simulink model "rst_auto_reg_test"  (R2019a)
settings: Solver=VariableStepAuto  StartTime=0.0  StopTime=150  RelTol=1e-3
values from neighbouring files (symbols this model uses):
  A = den    [cod_teste_RST_2.m]
  B = num    (= 1)    [cod_teste_RST_2.m]
  den = [10 1]    [cod_teste_RST_1.m]    (also in cod_teste_RST_2.m = [0.1 1.1 1])
  ep = 0.6    [cod_teste_RST_2.m]
  num = 1    [cod_teste_RST_1.m]    (also in cod_teste_RST_2.m)
  R = X(1)    [cod_teste_RST_1.m]    (also in cod_teste_RST_2.m = [X(1) X(2)])
  S = X(2:end)    [cod_teste_RST_1.m]    (also in cod_teste_RST_2.m = [X(3) X(4)])
  T = sum(PMF)/sum(B)    [cod_teste_RST_1.m]    (also in cod_teste_RST_2.m = sum(Am)/sum(B))
  Ta = 1    [cod_teste_RST_1.m]    (also in cod_teste_RST_2.m = 0.1)
  Ts = 1    [cod_teste_RST_2.m]
libraries: dspinverses x2
settings Model: Creator=Carlos Henrique  LastModifiedBy=PICHAU
settings DataIOCC: SaveOutput=off  SaveState=on  SignalLogging=off  DSMLogging=off  ReturnWorkspaceOutputs=off
settings DebuggingCC: ArithmeticOperatorsInVariantConditions=warning

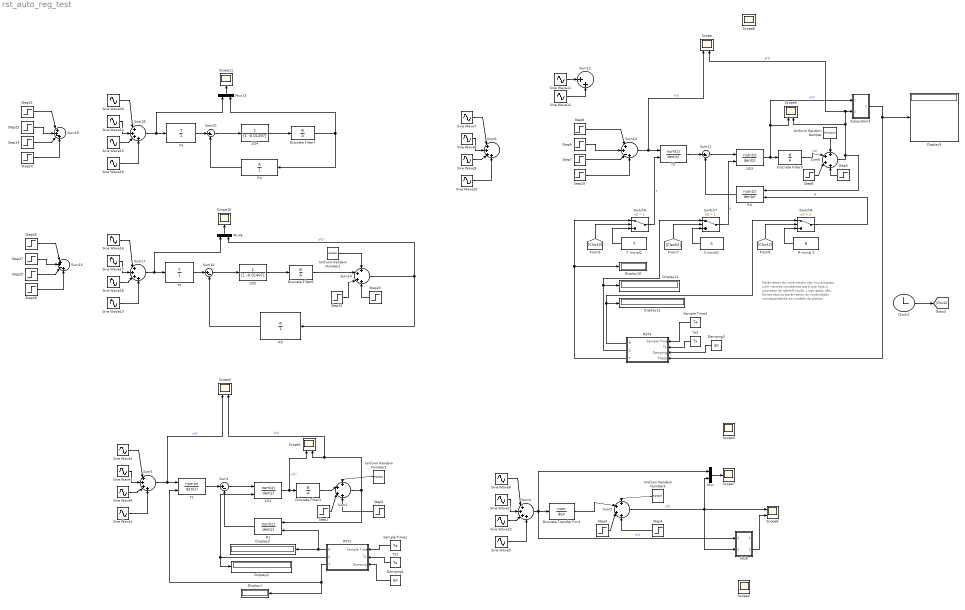
== system rst_auto_reg_test ==
  note: Parâmetros do controlador são inicializados
      | com valores constantes para que haja o
      | processo de identificação. Logo após, são
      | fornecidos os parâmetros do controlador
      | correspondente ao modelo da planta.
  1/S1 : DiscreteFilter  Numerator=1  DenominatorSource=Input port  Denominator=1  a0EqualsOne=on
      settings: InputPortMap=u0,p3
  1/S3 : DiscreteFilter  Numerator=1  DenominatorSource=Input port  Denominator=1  a0EqualsOne=on
      settings: InputPortMap=u0,p3
  1/S4 : DiscreteFilter  Numerator=1  Denominator=[1 -0.01497]  a0EqualsOne=on
  1/S5 : DiscreteFilter  Numerator=1  Denominator=[1 -0.01497]  a0EqualsOne=on
  Clock2 : Clock
  Damping1 : Constant  Value=ep
  Damping3 : Constant  Value=ep
  Discrete Transfer Fcn2 : DiscreteTransferFcn  Numerator=num  Denominator=den  SampleTime=Ta
  Discrete Filter{1,3,6..7} (4 alike) : DiscreteFilter  Numerator=B  Denominator=A  SampleTime=0.1  a0EqualsOne=on
  Display{1..3,9..12} (7 alike) : Display
  MQR : Subsystem
  Mux : Mux  Inputs=2
  Mux13 : Mux  Inputs=2
  Mux8 : Mux  Inputs=2
  R inicial 2 : Constant  Value=R
  R1 : DiscreteFilter  NumeratorSource=Input port  Numerator=[-620.2 131.3]  Denominator=1
      settings: InputPortMap=u0,p1
  R3 : DiscreteFilter  NumeratorSource=Input port  Numerator=[-620.2 131.3]  Denominator=1
      settings: InputPortMap=u0,p1
  R4 : DiscreteFilter  Numerator=R  Denominator=1
  R5 : DiscreteFilter  Numerator=R  Denominator=1
  RST1 : Subsystem
  RST3 : Subsystem
  S inicial2 : Constant  Value=S
  Sample Time1 : Constant  Value=Ta
  Sample Time3 : Constant  Value=Ta
  Scope{,1..2,4,6,8..9} (7 alike) : Scope  NumInputPorts=2
  Scope{3,7,10..11} (4 alike) : Scope
  Sine Wave{1,5,10,13,19} (5 alike) : Sin  Frequency=8  SampleTime=0
  Sine Wave{2,6..7,11,16,20} (6 alike) : Sin  SampleTime=0
  Sine Wave{3,8,12,14,17,21} (6 alike) : Sin  Frequency=2  SampleTime=0
  Sine Wave{4,9,15,18,22} (5 alike) : Sin  Frequency=4  SampleTime=0
  Step1 : Step  Time=50  SampleTime=0
  Step10 : Step  Time=30  SampleTime=0
  Step13 : Step  Time=50  SampleTime=0
  Step14 : Step  Time=20  After=2  SampleTime=0
  Step2 : Step  Time=51  After=-1  SampleTime=0
  Step21 : Step  Time=0  SampleTime=0
  Step22 : Step  Time=10  After=3  SampleTime=0
  Step23 : Step  Time=51  After=-1  SampleTime=0
  Step24 : Step  Time=30  SampleTime=0
  Step25 : Step  Time=20  After=2  SampleTime=0
  Step26 : Step  Time=0  SampleTime=0
  Step27 : Step  Time=10  After=3  SampleTime=0
  Step28 : Step  Time=30  SampleTime=0
  Step3 : Step  Time=50  SampleTime=0
  Step4 : Step  Time=51  After=-1  SampleTime=0
  Step5 : Step  Time=51  After=-0.2  SampleTime=0
  Step6 : Step  Time=50  After=0.2  SampleTime=0
  Step7 : Step  Time=20  After=2  SampleTime=0
  Step8 : Step  Time=0  SampleTime=0
  Step9 : Step  Time=10  After=3  SampleTime=0
  Subsystem3 : Subsystem
  Sum{1,11,16,20} (4 alike) : Sum  Inputs=|+-
  Sum10 : Sum  Inputs=|++-+
  Sum12 : Sum  Inputs=|++
  Sum{2,5..6,14} (4 alike) : Sum  Inputs=++++
  Sum15 : Sum  Inputs=|++-+
  Sum{3..4,9,17..18} (5 alike) : Sum  Inputs=|++++
  Sum19 : Sum  Inputs=|++-+
  Switch6 : Switch  Criteria=u2 > Threshold  Threshold=1
  Switch7 : Switch  Criteria=u2 > Threshold  Threshold=1
  Switch8 : Switch  Criteria=u2 > Threshold  Threshold=1
  T inicial2 : Constant  Value=T
  T1 : DiscreteFilter  NumeratorSource=Input port  Numerator=13.39  Denominator=1
      settings: InputPortMap=u0,p1
  T3 : DiscreteFilter  NumeratorSource=Input port  Numerator=13.39  Denominator=1
      settings: InputPortMap=u0,p1
  T4 : DiscreteFilter  Numerator=T  Denominator=1  a0EqualsOne=on
  T5 : DiscreteFilter  Numerator=T  Denominator=1  a0EqualsOne=on
  Ts1 : Constant  Value=Ts
  Ts3 : Constant  Value=Ts
  Uniform Random Number : UniformRandomNumber  Minimum=-0.01  Maximum=0.01  SampleTime=0
  Uniform Random Number1 : UniformRandomNumber  Minimum=-0.1  Maximum=0.1  SampleTime=0
  Uniform Random Number2 : UniformRandomNumber  Minimum=-0.1  Maximum=0.1  SampleTime=0
  Uniform Random Number3 : UniformRandomNumber  Minimum=-0.01  Maximum=0.01  SampleTime=0
  wires:
  Sine Wave10/1 -> Sum9/4
  Ts3/1 -> RST3/2(Ts)
  T3/1 -> Sum11/1
  R3/1 -> Sum11/2
  RST3/1(R) -> Switch8/1, Display12/1
  Switch8/1 -> R3/2  "R"
  Step7/1 -> Sum10/3
  RST3/2(S) -> Switch7/1, Display11/1
  [Clock2] -> Switch7/2
  Subsystem3/1(Out1) -> RST3/4(Theta), Display9/1
  T inicial2/1 -> Switch6/3
  Sine Wave7/1 -> Sum9/1
  Clock2/1 -> [Clock2]
  S inicial2/1 -> Switch7/3
  Sum11/1 -> 1/S3/1
  Switch6/1 -> T3/2  "T"
  [Clock2] -> Switch6/2
  Switch7/1 -> 1/S3/2  "S"
  Sample Time3/1 -> RST3/1(Sample Time)
  Sine Wave8/1 -> Sum9/2
  Damping3/1 -> RST3/3(Damping)
  RST3/3(T) -> Switch6/1, Display10/1
  R inicial 2/1 -> Switch8/3
  Sine Wave9/1 -> Sum9/3
  Step9/1 -> Sum10/2
  Step8/1 -> Sum10/1
  Step10/1 -> Sum10/4
  1/S3/1 -> Scope9/1, Subsystem3/1(In1), Discrete Filter3/1  "u(t)"
  [Clock2] -> Switch8/2
  Sine Wave12/1 -> Sum12/2
  Sine Wave11/1 -> Sum12/1
  Sum10/1 -> Scope/1, T3/1  "r(t)"
  Sum17/1 -> Mux8/1, T5/1
  Sum18/1 -> Mux13/1, T4/1
  Sine Wave19/1 -> Sum18/4
  Step13/1 -> Sum14/3
  Uniform Random Number1/1 -> Sum14/1
  Sine Wave15/1 -> Sum18/3
  Step14/1 -> Sum19/3
  Step24/1 -> Sum19/4
  Step21/1 -> Sum19/1
  Step23/1 -> Sum14/4
  Sum20/1 -> 1/S4/1
  T4/1 -> Sum20/1
  1/S5/1 -> Discrete Filter6/1
  Step27/1 -> Sum15/2
  Step22/1 -> Sum19/2
  1/S4/1 -> Discrete Filter7/1
  R5/1 -> Sum16/2
  Sine Wave20/1 -> Sum18/1
  Sine Wave16/1 -> Sum17/1
  Sine Wave17/1 -> Sum17/2
  Sum14/1 -> R5/1, Mux8/2  "y(t)"
  Step25/1 -> Sum15/3
  Sine Wave18/1 -> Sum17/3
  Sine Wave13/1 -> Sum17/4
  Discrete Filter6/1 -> Sum14/2
  Mux13/1 -> Scope11/1
  Sum16/1 -> 1/S5/1
  Discrete Filter7/1 -> R4/1, Mux13/2
  Sine Wave14/1 -> Sum18/2
  Step26/1 -> Sum15/1
  R4/1 -> Sum20/2
  Mux8/1 -> Scope10/1
  Step28/1 -> Sum15/4
  T5/1 -> Sum16/1
  1/S1/1 -> Scope1/1, Discrete Filter1/1  "u(t)"
  RST1/3(T) -> T1/2, Display1/1
  Sine Wave4/1 -> Sum3/3
  Sum2/1 -> R1/1, Scope2/2, Scope1/2  "y(t)"
  Sine Wave1/1 -> Sum3/4
  Damping1/1 -> RST1/3(Damping)
  Sum1/1 -> 1/S1/1
  T1/1 -> Sum1/1
  RST1/1(R) -> R1/2, Display3/1
  Discrete Filter1/1 -> Sum2/2
  Ts1/1 -> RST1/2(Ts)
  Sample Time1/1 -> RST1/1(Sample Time)
  Step1/1 -> Sum2/3
  Sine Wave2/1 -> Sum3/1
  Step2/1 -> Sum2/4
  Sum3/1 -> Scope2/1, T1/1  "r(t)"
  RST1/2(S) -> Display2/1, 1/S1/2
  Uniform Random Number2/1 -> Sum2/1
  R1/1 -> Sum1/2
  Sine Wave3/1 -> Sum3/2
  Mux/1 -> Scope7/1
  Sum4/1 -> Mux/1, MQR/1(In1), Discrete Transfer Fcn2/1  "r(t)"
  Sine Wave21/1 -> Sum4/2
  Sine Wave6/1 -> Sum4/1
  Sine Wave5/1 -> Sum4/4
  Sine Wave22/1 -> Sum4/3
  Uniform Random Number3/1 -> Sum5/1
  Sum5/1 -> Scope6/1, Mux/2, MQR/2(In2)  "y(t)"
  Step3/1 -> Sum5/3
  Step4/1 -> Sum5/4
  Discrete Transfer Fcn2/1 -> Sum5/2
  Step5/1 -> Sum6/4
  Step6/1 -> Sum6/3
  Discrete Filter3/1 -> Sum6/2  "y(t)"
  Sum6/1 -> R3/1, Scope9/2, Scope/2, Subsystem3/2(In2)  "y(t)"
  Uniform Random Number/1 -> Sum6/1
  MQR/2(Out2) -> Scope6/2

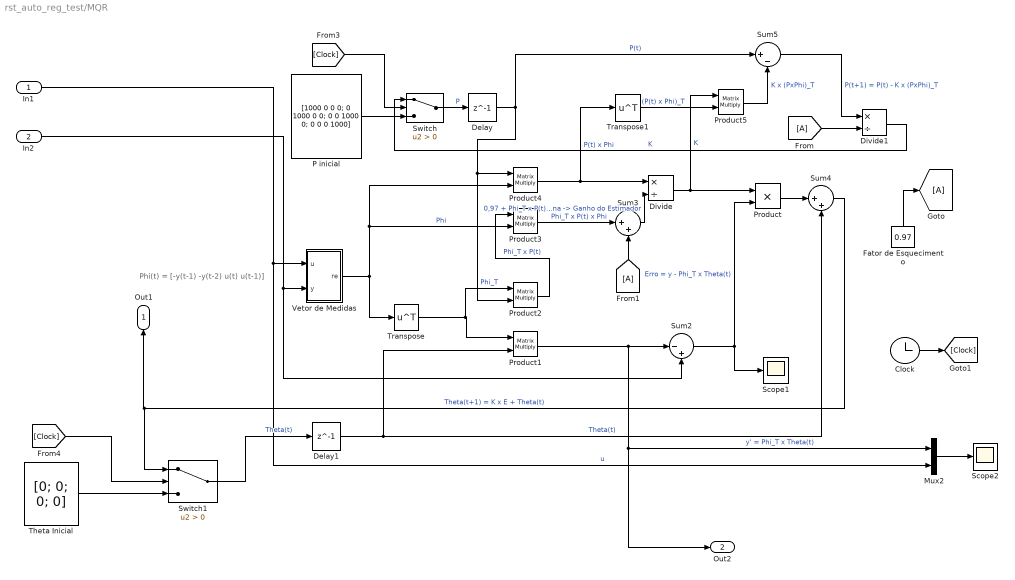
== system rst_auto_reg_test/MQR ==
  note: Phi(t) = [-y(t-1) -y(t-2) u(t) u(t-1)]
  In1 : Inport
  In2 : Inport  Port=2
  Clock : Clock
  Delay : Delay  DelayLength=1  InitialCondition=0  SampleTime=0.1
  Delay1 : Delay  DelayLength=1  InitialCondition=0  SampleTime=0.1
  Divide : Product  Inputs=*/
  Divide1 : Product  Inputs=*/
  "Fator de Esquecimento " : Constant  Value=0.97
  Mux2 : Mux  Inputs=2
  P inicial : Constant  Value=[1000 0 0 0; 0 1000 0 0; 0 0 1000 0; 0 0 0 1000]
  Product : Product
  Product{1..5} (5 alike) : Product  Multiplication=Matrix(*)
  Scope1 : Scope
  Scope2 : Scope
  Sum2 : Sum  Inputs=|-+
  Sum3 : Sum  Inputs=|++
  Sum4 : Sum  Inputs=|++
  Sum5 : Sum  Inputs=|+-
  Switch : Switch  Criteria=u2 > Threshold
  Switch1 : Switch  Criteria=u2 > Threshold
  "Theta Inicial " : Constant  Value=[0; 0; 0; 0]
  Transpose : Math  Operator=transpose  SaturateOnIntegerOverflow=on
  Transpose1 : Math  Operator=transpose  SaturateOnIntegerOverflow=on
  "Vetor de Medidas " : Subsystem
  Out1 : Outport
  Out2 : Outport  Port=2
  wires:
  "Vetor de Medidas "/1(re) -> Transpose/1, Product4/2, Product3/2  "Phi"
  Product/1 -> Sum4/1
  In2/1 -> "Vetor de Medidas "/2(y), Sum2/2
  "Fator de Esquecimento "/1 -> [A]
  Transpose/1 -> Product2/1, Product1/1  "Phi_T"
  Sum3/1 -> Divide/2  "0,97 + Phi_T x P(t) x Phi Vetor Coluna -> Ganho do Estimador"
  Product3/1 -> Sum3/1  "Phi_T x P(t) x Phi"
  Switch/1 -> Delay/1  "P"
  Product4/1 -> Transpose1/1, Divide/1  "P(t) x Phi"
  Delay/1 -> Product4/1, Product2/2, Sum5/1  "P(t)"
  Divide/1 -> Product5/1, Product/1  "K"
  Transpose1/1 -> Product5/2  "(P(t) x Phi)_T"
  Sum5/1 -> Divide1/1  "P(t+1) = P(t) - K x (PxPhi)_T"
  Sum2/1 -> Scope1/1, Product/2  "Erro = y - Phi_T x Theta(t)"
  Delay1/1 -> Sum4/2, Product1/2  "Theta(t)"
  Divide1/1 -> Switch/1  "K"
  "Theta Inicial "/1 -> Switch1/3
  [A] -> Divide1/2
  Product2/1 -> Product3/1  "Phi_T x P(t)"
  Clock/1 -> [Clock]
  Product1/1 -> Out2/1, Mux2/1, Sum2/1  "y' = Phi_T x Theta(t)"
  Product5/1 -> Sum5/2  "K x (PxPhi)_T"
  P inicial/1 -> Switch/3
  Sum4/1 -> Switch1/1, Out1/1  "Theta(t+1) = K x E + Theta(t)"
  [A] -> Sum3/2
  In1/1 -> "Vetor de Medidas "/1(u), Mux2/2  "u"
  [Clock] -> Switch/2
  Switch1/1 -> Delay1/1  "Theta(t)"
  Mux2/1 -> Scope2/1
  [Clock] -> Switch1/2

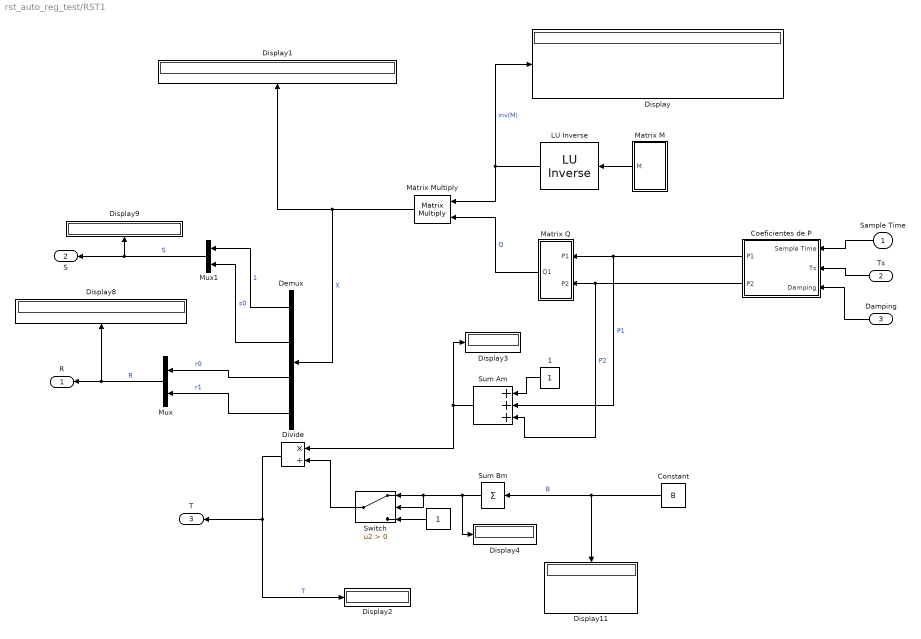
== system rst_auto_reg_test/RST1 ==
  Sample Time : Inport
  Ts : Inport  Port=2
  Damping : Inport  Port=3
  " " : Constant
  " LU Inverse" : dspinverses/ LU Inverse
      settings: SourceProductName=DSP System Toolbox
  1 : Constant
  Coeficientes de P : Subsystem
  Constant : Constant  Value=B
  Demux : Demux
  Display{,1..4,8..9,11} (8 alike) : Display
  Divide : Product  Inputs=*/
  Matrix M : Subsystem
  Matrix Multiply : Product  Multiplication=Matrix(*)
  Matrix Q : Subsystem
  Mux : Mux  Inputs=2
  Mux1 : Mux  Inputs=2
  Sum Am : Sum  Inputs=+++
  Sum Bm : Sum  Inputs=+
  Switch : Switch  Criteria=u2 > Threshold
  R : Outport
  S : Outport  Port=2
  T : Outport  Port=3
  wires:
  Matrix Multiply/1 -> Demux/1, Display1/1  "X"
  Sum Bm/1 -> Switch/2, Switch/1, Display4/1
  " LU Inverse"/1 -> Matrix Multiply/1, Display/1  "inv(M)"
  Sum Am/1 -> Divide/1, Display3/1
  Mux1/1 -> S/1, Display9/1  "S"
  Coeficientes de P/2(P2) -> Matrix Q/2(P2), Sum Am/3  "P2"
  Divide/1 -> T/1, Display2/1  "T"
  Ts/1 -> Coeficientes de P/2(Ts)
  Damping/1 -> Coeficientes de P/3(Damping)
  Sample Time/1 -> Coeficientes de P/1(Sample Time)
  1/1 -> Sum Am/1
  Coeficientes de P/1(P1) -> Matrix Q/1(P1), Sum Am/2  "P1"
  Constant/1 -> Display11/1, Sum Bm/1  "B"
  Switch/1 -> Divide/2
  " "/1 -> Switch/3
  Mux/1 -> R/1, Display8/1  "R"
  Matrix M/1(M) -> " LU Inverse"/1
  Matrix Q/1(Q1) -> Matrix Multiply/2  "Q"
  Demux/1 -> Mux1/1  "1"
  Demux/2 -> Mux1/2  "s0"
  Demux/3 -> Mux/1  "r0"
  Demux/4 -> Mux/2  "r1"

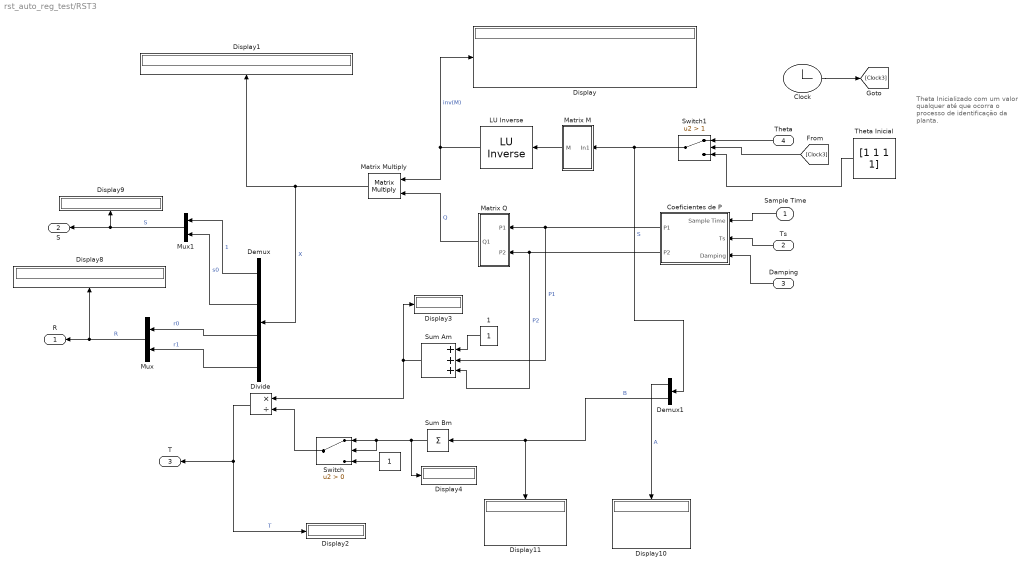
== system rst_auto_reg_test/RST3 ==
  note: Theta Inicializado com um
      | valor qualquer até que ocorra
      |  o processo de identificação
      | da planta.
  Sample Time : Inport
  Ts : Inport  Port=2
  Damping : Inport  Port=3
  Theta : Inport  Port=4
  " " : Constant
  " LU Inverse" : dspinverses/ LU Inverse
      settings: SourceProductName=DSP System Toolbox
  1 : Constant
  Clock : Clock
  Coeficientes de P : Subsystem
  Demux : Demux
  Demux1 : Demux  Outputs=2
  Display{,1..4,8..11} (9 alike) : Display
  Divide : Product  Inputs=*/
  Matrix M : Subsystem
  Matrix Multiply : Product  Multiplication=Matrix(*)
  Matrix Q : Subsystem
  Mux : Mux  Inputs=2
  Mux1 : Mux  Inputs=2
  Sum Am : Sum  Inputs=+++
  Sum Bm : Sum  Inputs=+
  Switch : Switch  Criteria=u2 > Threshold
  Switch1 : Switch  Criteria=u2 > Threshold  Threshold=1
  Theta Inicial : Constant  Value=[1 1 1 1]
  R : Outport
  S : Outport  Port=2
  T : Outport  Port=3
  wires:
  Matrix Multiply/1 -> Demux/1, Display1/1  "X"
  Sum Bm/1 -> Switch/2, Switch/1, Display4/1
  " LU Inverse"/1 -> Matrix Multiply/1, Display/1  "inv(M)"
  Sum Am/1 -> Divide/1, Display3/1
  Mux1/1 -> S/1, Display9/1  "S"
  Coeficientes de P/2(P2) -> Matrix Q/2(P2), Sum Am/3  "P2"
  Divide/1 -> T/1, Display2/1  "T"
  Ts/1 -> Coeficientes de P/2(Ts)
  Damping/1 -> Coeficientes de P/3(Damping)
  Sample Time/1 -> Coeficientes de P/1(Sample Time)
  1/1 -> Sum Am/1
  Coeficientes de P/1(P1) -> Matrix Q/1(P1), Sum Am/2  "P1"
  Demux1/2 -> Display11/1, Sum Bm/1  "B"
  Demux1/1 -> Display10/1  "A"
  Switch/1 -> Divide/2
  " "/1 -> Switch/3
  Mux/1 -> R/1, Display8/1  "R"
  Clock/1 -> [Clock3]
  Switch1/1 -> Matrix M/1(In1), Demux1/1  "S"
  Theta/1 -> Switch1/1
  [Clock3] -> Switch1/2
  Theta Inicial/1 -> Switch1/3
  Matrix M/1(M) -> " LU Inverse"/1
  Matrix Q/1(Q1) -> Matrix Multiply/2  "Q"
  Demux/1 -> Mux1/1  "1"
  Demux/2 -> Mux1/2  "s0"
  Demux/3 -> Mux/1  "r0"
  Demux/4 -> Mux/2  "r1"

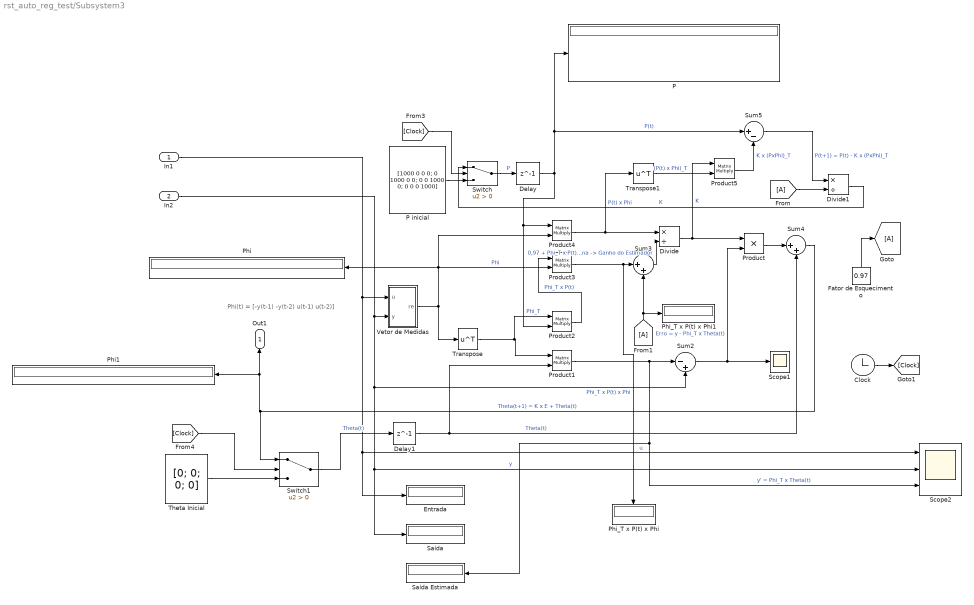
== system rst_auto_reg_test/Subsystem3 ==
  note: Phi(t) = [-y(t-1) -y(t-2) u(t-1) u(t-2)]
  In1 : Inport
  In2 : Inport  Port=2
  Clock : Clock
  Delay : Delay  DelayLength=1  InitialCondition=0  SampleTime=0.1
  Delay1 : Delay  DelayLength=1  InitialCondition=0  SampleTime=0.1
  Divide : Product  Inputs=*/
  Divide1 : Product  Inputs=*/
  Entrada : Display
  "Fator de Esquecimento " : Constant  Value=0.97
  P : Display
  P inicial : Constant  Value=[1000 0 0 0; 0 1000 0 0; 0 0 1000 0; 0 0 0 1000]
  Phi : Display
  Phi1 : Display
  Phi_T x P(t) x Phi : Display
  Phi_T x P(t) x Phi1 : Display
  Product : Product
  Product{1..5} (5 alike) : Product  Multiplication=Matrix(*)
  Saída : Display
  "Saída Estimada " : Display
  Scope1 : Scope
  Scope2 : Scope  NumInputPorts=3
  Sum2 : Sum  Inputs=|-+
  Sum3 : Sum  Inputs=|++
  Sum4 : Sum  Inputs=|++
  Sum5 : Sum  Inputs=|+-
  Switch : Switch  Criteria=u2 > Threshold
  Switch1 : Switch  Criteria=u2 > Threshold
  "Theta Inicial " : Constant  Value=[0; 0; 0; 0]
  Transpose : Math  Operator=transpose  SaturateOnIntegerOverflow=on
  Transpose1 : Math  Operator=transpose  SaturateOnIntegerOverflow=on
  "Vetor de Medidas " : Subsystem
  Out1 : Outport
  wires:
  "Vetor de Medidas "/1(re) -> Product4/2, Phi/1, Product3/2, Transpose/1  "Phi"
  Product/1 -> Sum4/1
  In2/1 -> Saída/1, Scope2/2, Sum2/2, "Vetor de Medidas "/2(y)  "y"
  "Fator de Esquecimento "/1 -> [A]
  Transpose/1 -> Product2/1, Product1/1  "Phi_T"
  Sum3/1 -> Divide/2  "0,97 + Phi_T x P(t) x Phi Vetor Coluna -> Ganho do Estimador"
  Product3/1 -> Phi_T x P(t) x Phi/1, Sum3/1  "Phi_T x P(t) x Phi"
  Switch/1 -> Delay/1  "P"
  Product4/1 -> Transpose1/1, Divide/1  "P(t) x Phi"
  Delay/1 -> Product2/2, Product4/1, P/1, Sum5/1  "P(t)"
  Divide/1 -> Product5/1, Product/1  "K"
  Transpose1/1 -> Product5/2  "(P(t) x Phi)_T"
  Sum5/1 -> Divide1/1  "P(t+1) = P(t) - K x (PxPhi)_T"
  Sum2/1 -> Scope1/1, Product/2  "Erro = y - Phi_T x Theta(t)"
  Delay1/1 -> Sum4/2, Product1/2  "Theta(t)"
  Divide1/1 -> Switch/1  "K"
  "Theta Inicial "/1 -> Switch1/3
  [A] -> Divide1/2
  Product2/1 -> Product3/1  "Phi_T x P(t)"
  Clock/1 -> [Clock]
  Product1/1 -> Sum2/1, Scope2/3, "Saída Estimada "/1  "y' = Phi_T x Theta(t)"
  Product5/1 -> Sum5/2  "K x (PxPhi)_T"
  P inicial/1 -> Switch/3
  Sum4/1 -> Switch1/1, Phi1/1, Out1/1  "Theta(t+1) = K x E + Theta(t)"
  [A] -> Sum3/2, Phi_T x P(t) x Phi1/1
  In1/1 -> Entrada/1, Scope2/1, "Vetor de Medidas "/1(u)  "u"
  [Clock] -> Switch/2
  Switch1/1 -> Delay1/1  "Theta(t)"
  [Clock] -> Switch1/2

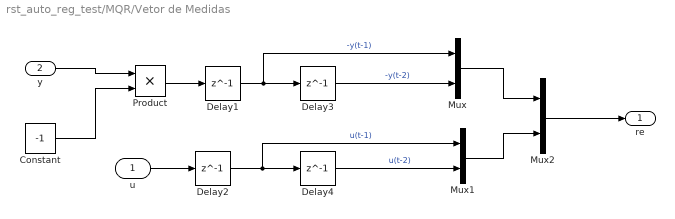
== system rst_auto_reg_test/MQR/Vetor de Medidas  ==
  u : Inport
  y : Inport  Port=2
  Constant : Constant  Value=-1
  Delay{1..4} (4 alike) : Delay  DelayLength=1  InitialCondition=0  SampleTime=0.1
  Mux : Mux  Inputs=2
  Mux1 : Mux  Inputs=2
  Mux2 : Mux  Inputs=2
  Product : Product
  re : Outport
  wires:
  u/1 -> Delay2/1
  Mux/1 -> Mux2/1
  Product/1 -> Delay1/1
  Delay2/1 -> Mux1/1, Delay4/1  "u(t-1)"
  Delay3/1 -> Mux/2  "-y(t-2)"
  Constant/1 -> Product/2
  Mux2/1 -> re/1
  y/1 -> Product/1
  Delay1/1 -> Mux/1, Delay3/1  "-y(t-1)"
  Delay4/1 -> Mux1/2  "u(t-2)"
  Mux1/1 -> Mux2/2

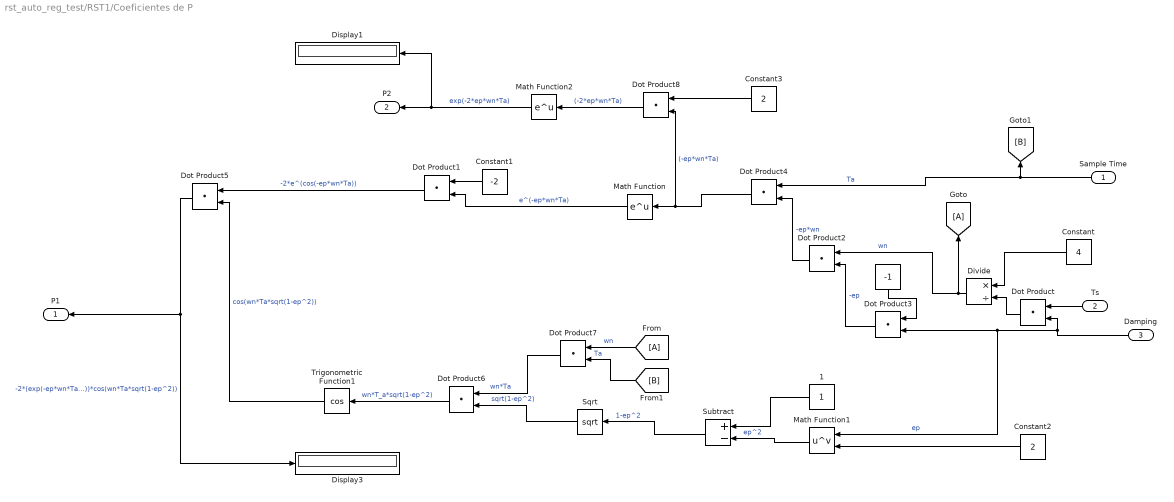
== system rst_auto_reg_test/RST1/Coeficientes de P ==
  Sample Time : Inport
  Ts : Inport  Port=2
  Damping : Inport  Port=3
  " " : Constant  Value=-1
  1 : Constant
  Constant : Constant  Value=4
  Constant1 : Constant  Value=-2
  Constant2 : Constant  Value=2
  Constant3 : Constant  Value=2
  Display1 : Display
  Display3 : Display
  Divide : Product  Inputs=*/
  Dot Product{,1..8} (9 alike) : DotProduct  InputSameDT=on  OutDataTypeStr=Inherit: Inherit via internal rule
  Math Function : Math  SaturateOnIntegerOverflow=on
  Math Function1 : Math  Operator=pow  SaturateOnIntegerOverflow=on
  Math Function2 : Math  SaturateOnIntegerOverflow=on
  Sqrt : Sqrt  SaturateOnIntegerOverflow=on
  Subtract : Sum  Inputs=+-
  Trigonometric Function1 : Trigonometry  Operator=cos
  P1 : Outport
  P2 : Outport  Port=2
  wires:
  Math Function/1 -> Dot Product1/2  "e^(-ep*wn*Ta)"
  Divide/1 -> [A], Dot Product2/1  "wn"
  [A] -> Dot Product7/1  "wn"
  " "/1 -> Dot Product3/1
  Dot Product5/1 -> P1/1, Display3/1  "-2*(exp(-ep*wn*Ta))*cos(wn*Ta*sqrt(1-ep^2))"
  Trigonometric Function1/1 -> Dot Product5/2  "cos(wn*Ta*sqrt(1-ep^2))"
  Ts/1 -> Dot Product/1
  Dot Product/1 -> Divide/2
  Dot Product3/1 -> Dot Product2/2  "-ep"
  Damping/1 -> Math Function1/1, Dot Product3/2, Dot Product/2  "ep"
  Constant/1 -> Divide/1
  Dot Product7/1 -> Dot Product6/1  "wn*Ta"
  Sample Time/1 -> Dot Product4/1, [B]  "Ta"
  Math Function1/1 -> Subtract/2  "ep^2"
  Dot Product1/1 -> Dot Product5/1  "-2*e^(cos(-ep*wn*Ta))"
  Constant2/1 -> Math Function1/2
  1/1 -> Subtract/1
  Constant1/1 -> Dot Product1/1
  Dot Product2/1 -> Dot Product4/2  "-ep*wn"
  [B] -> Dot Product7/2  "Ta"
  Dot Product6/1 -> Trigonometric Function1/1  "wn*T_a*sqrt(1-ep^2)"
  Dot Product4/1 -> Dot Product8/2, Math Function/1  "(-ep*wn*Ta)"
  Sqrt/1 -> Dot Product6/2  "sqrt(1-ep^2)"
  Subtract/1 -> Sqrt/1  "1-ep^2"
  Constant3/1 -> Dot Product8/1
  Dot Product8/1 -> Math Function2/1  "(-2*ep*wn*Ta)"
  Math Function2/1 -> Display1/1, P2/1  "exp(-2*ep*wn*Ta)"

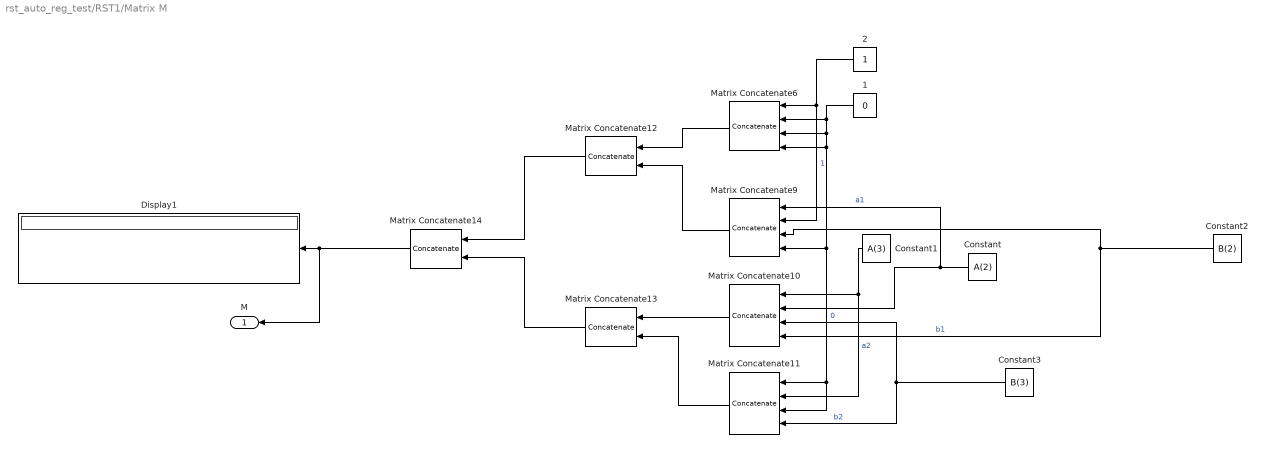
== system rst_auto_reg_test/RST1/Matrix M ==
  " 1" : Constant  Value=0
  2 : Constant
  Constant : Constant  Value=A(2)
  Constant1 : Constant  Value=A(3)
  Constant2 : Constant  Value=B(2)
  Constant3 : Constant  Value=B(3)
  Display1 : Display
  Matrix Concatenate{6,9..11} (4 alike) : Concatenate  NumInputs=4  Mode=Multidimensional array  ConcatenateDimension=2
  Matrix Concatenate12 : Concatenate  Mode=Multidimensional array
  Matrix Concatenate13 : Concatenate  Mode=Multidimensional array
  Matrix Concatenate14 : Concatenate  Mode=Multidimensional array
  M : Outport
  wires:
  Constant2/1 -> Matrix Concatenate9/3, Matrix Concatenate10/4  "b1"
  Matrix Concatenate14/1 -> M/1, Display1/1
  Constant/1 -> Matrix Concatenate9/1, Matrix Concatenate10/2  "a1"
  Constant3/1 -> Matrix Concatenate10/3, Matrix Concatenate11/4  "b2"
  Constant1/1 -> Matrix Concatenate11/2, Matrix Concatenate10/1  "a2"
  2/1 -> Matrix Concatenate9/2, Matrix Concatenate6/1  "1"
  " 1"/1 -> Matrix Concatenate6/3, Matrix Concatenate11/3, Matrix Concatenate11/1, Matrix Concatenate9/4, Matrix Concatenate6/4, Matrix Concatenate6/2  "0"
  Matrix Concatenate6/1 -> Matrix Concatenate12/1
  Matrix Concatenate9/1 -> Matrix Concatenate12/2
  Matrix Concatenate10/1 -> Matrix Concatenate13/1
  Matrix Concatenate11/1 -> Matrix Concatenate13/2
  Matrix Concatenate13/1 -> Matrix Concatenate14/2
  Matrix Concatenate12/1 -> Matrix Concatenate14/1

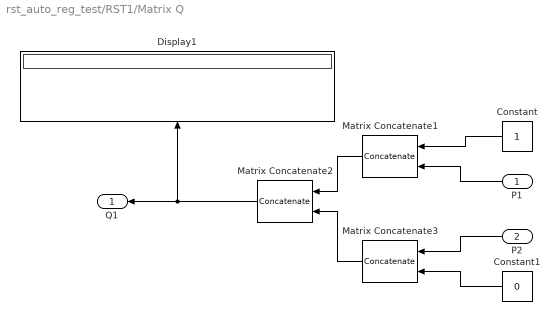
== system rst_auto_reg_test/RST1/Matrix Q ==
  P1 : Inport
  P2 : Inport  Port=2
  Constant : Constant
  Constant1 : Constant  Value=0
  Display1 : Display
  Matrix Concatenate1 : Concatenate  Mode=Multidimensional array
  Matrix Concatenate2 : Concatenate  Mode=Multidimensional array
  Matrix Concatenate3 : Concatenate  Mode=Multidimensional array
  Q1 : Outport
  wires:
  Matrix Concatenate1/1 -> Matrix Concatenate2/1
  Matrix Concatenate2/1 -> Q1/1, Display1/1
  Matrix Concatenate3/1 -> Matrix Concatenate2/2
  P2/1 -> Matrix Concatenate3/1
  P1/1 -> Matrix Concatenate1/2
  Constant/1 -> Matrix Concatenate1/1
  Constant1/1 -> Matrix Concatenate3/2

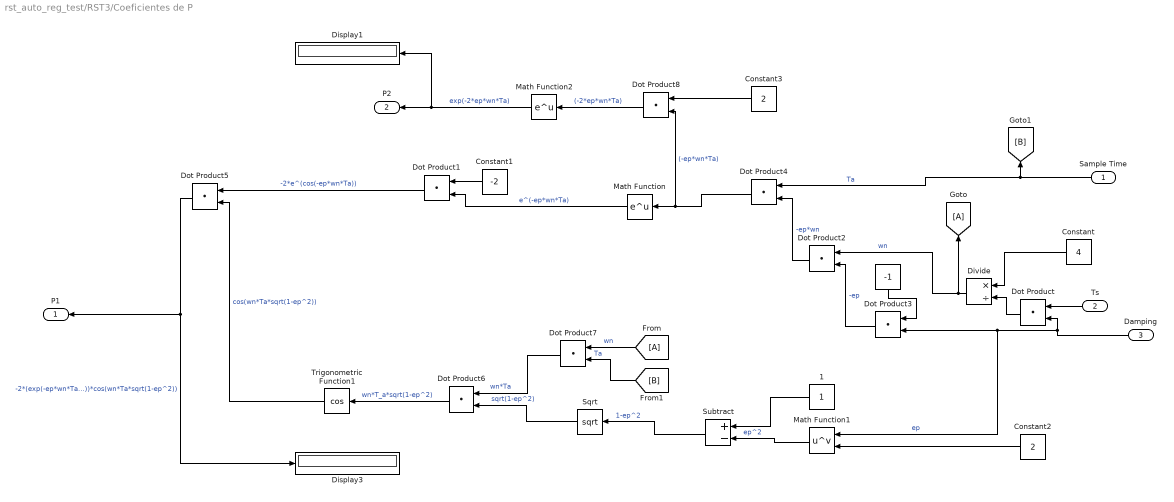
== system rst_auto_reg_test/RST3/Coeficientes de P ==
  Sample Time : Inport
  Ts : Inport  Port=2
  Damping : Inport  Port=3
  " " : Constant  Value=-1
  1 : Constant
  Constant : Constant  Value=4
  Constant1 : Constant  Value=-2
  Constant2 : Constant  Value=2
  Constant3 : Constant  Value=2
  Display1 : Display
  Display3 : Display
  Divide : Product  Inputs=*/
  Dot Product{,1..8} (9 alike) : DotProduct  InputSameDT=on  OutDataTypeStr=Inherit: Inherit via internal rule
  Math Function : Math  SaturateOnIntegerOverflow=on
  Math Function1 : Math  Operator=pow  SaturateOnIntegerOverflow=on
  Math Function2 : Math  SaturateOnIntegerOverflow=on
  Sqrt : Sqrt  SaturateOnIntegerOverflow=on
  Subtract : Sum  Inputs=+-
  Trigonometric Function1 : Trigonometry  Operator=cos
  P1 : Outport
  P2 : Outport  Port=2
  wires:
  Math Function/1 -> Dot Product1/2  "e^(-ep*wn*Ta)"
  Divide/1 -> [A], Dot Product2/1  "wn"
  [A] -> Dot Product7/1  "wn"
  " "/1 -> Dot Product3/1
  Dot Product5/1 -> P1/1, Display3/1  "-2*(exp(-ep*wn*Ta))*cos(wn*Ta*sqrt(1-ep^2))"
  Trigonometric Function1/1 -> Dot Product5/2  "cos(wn*Ta*sqrt(1-ep^2))"
  Ts/1 -> Dot Product/1
  Dot Product/1 -> Divide/2
  Dot Product3/1 -> Dot Product2/2  "-ep"
  Damping/1 -> Math Function1/1, Dot Product3/2, Dot Product/2  "ep"
  Constant/1 -> Divide/1
  Dot Product7/1 -> Dot Product6/1  "wn*Ta"
  Sample Time/1 -> Dot Product4/1, [B]  "Ta"
  Math Function1/1 -> Subtract/2  "ep^2"
  Dot Product1/1 -> Dot Product5/1  "-2*e^(cos(-ep*wn*Ta))"
  Constant2/1 -> Math Function1/2
  1/1 -> Subtract/1
  Constant1/1 -> Dot Product1/1
  Dot Product2/1 -> Dot Product4/2  "-ep*wn"
  [B] -> Dot Product7/2  "Ta"
  Dot Product6/1 -> Trigonometric Function1/1  "wn*T_a*sqrt(1-ep^2)"
  Dot Product4/1 -> Dot Product8/2, Math Function/1  "(-ep*wn*Ta)"
  Sqrt/1 -> Dot Product6/2  "sqrt(1-ep^2)"
  Subtract/1 -> Sqrt/1  "1-ep^2"
  Constant3/1 -> Dot Product8/1
  Dot Product8/1 -> Math Function2/1  "(-2*ep*wn*Ta)"
  Math Function2/1 -> Display1/1, P2/1  "exp(-2*ep*wn*Ta)"

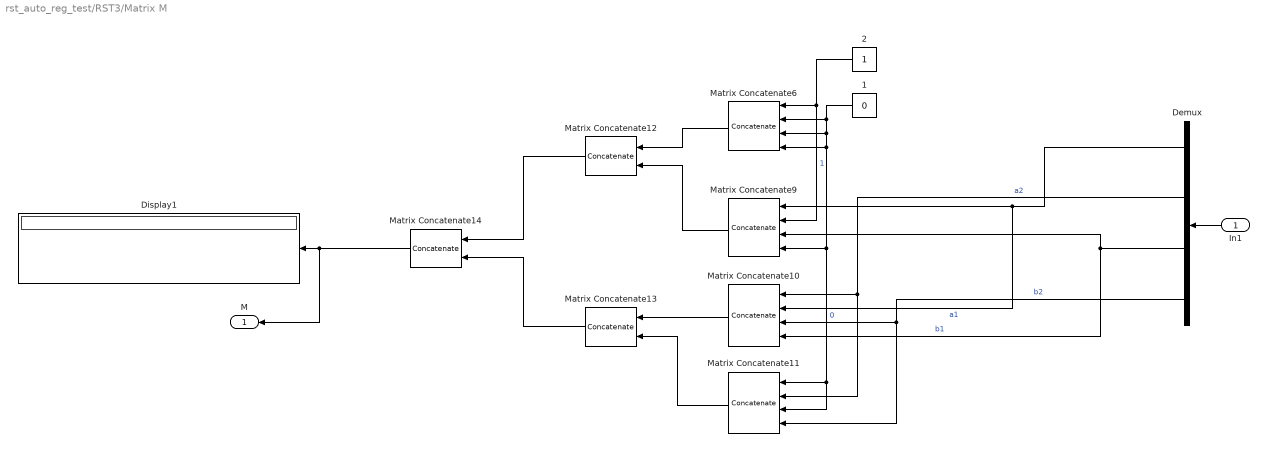
== system rst_auto_reg_test/RST3/Matrix M ==
  In1 : Inport
  " 1" : Constant  Value=0
  2 : Constant
  Demux : Demux
  Display1 : Display
  Matrix Concatenate{6,9..11} (4 alike) : Concatenate  NumInputs=4  Mode=Multidimensional array  ConcatenateDimension=2
  Matrix Concatenate12 : Concatenate  Mode=Multidimensional array
  Matrix Concatenate13 : Concatenate  Mode=Multidimensional array
  Matrix Concatenate14 : Concatenate  Mode=Multidimensional array
  M : Outport
  wires:
  In1/1 -> Demux/1
  Demux/3 -> Matrix Concatenate9/3, Matrix Concatenate10/4  "b1"
  Matrix Concatenate14/1 -> M/1, Display1/1
  Demux/1 -> Matrix Concatenate10/2, Matrix Concatenate9/1  "a1"
  Demux/4 -> Matrix Concatenate11/4, Matrix Concatenate10/3  "b2"
  Demux/2 -> Matrix Concatenate11/2, Matrix Concatenate10/1  "a2"
  2/1 -> Matrix Concatenate9/2, Matrix Concatenate6/1  "1"
  " 1"/1 -> Matrix Concatenate6/3, Matrix Concatenate11/3, Matrix Concatenate11/1, Matrix Concatenate9/4, Matrix Concatenate6/4, Matrix Concatenate6/2  "0"
  Matrix Concatenate6/1 -> Matrix Concatenate12/1
  Matrix Concatenate9/1 -> Matrix Concatenate12/2
  Matrix Concatenate10/1 -> Matrix Concatenate13/1
  Matrix Concatenate11/1 -> Matrix Concatenate13/2
  Matrix Concatenate13/1 -> Matrix Concatenate14/2
  Matrix Concatenate12/1 -> Matrix Concatenate14/1

== system rst_auto_reg_test/RST3/Matrix Q ==
  P1 : Inport
  P2 : Inport  Port=2
  Constant : Constant
  Constant1 : Constant  Value=0
  Display1 : Display
  Matrix Concatenate1 : Concatenate  Mode=Multidimensional array
  Matrix Concatenate2 : Concatenate  Mode=Multidimensional array
  Matrix Concatenate3 : Concatenate  Mode=Multidimensional array
  Q1 : Outport
  wires:
  Matrix Concatenate1/1 -> Matrix Concatenate2/1
  Matrix Concatenate2/1 -> Q1/1, Display1/1
  Matrix Concatenate3/1 -> Matrix Concatenate2/2
  P2/1 -> Matrix Concatenate3/1
  P1/1 -> Matrix Concatenate1/2
  Constant/1 -> Matrix Concatenate1/1
  Constant1/1 -> Matrix Concatenate3/2

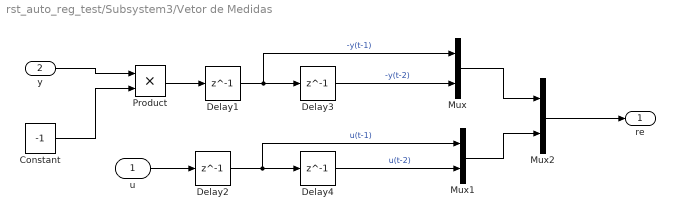
== system rst_auto_reg_test/Subsystem3/Vetor de Medidas  ==
  u : Inport
  y : Inport  Port=2
  Constant : Constant  Value=-1
  Delay{1..4} (4 alike) : Delay  DelayLength=1  InitialCondition=0  SampleTime=0.1
  Mux : Mux  Inputs=2
  Mux1 : Mux  Inputs=2
  Mux2 : Mux  Inputs=2
  Product : Product
  re : Outport
  wires:
  Delay4/1 -> Mux1/2  "u(t-2)"
  Mux1/1 -> Mux2/2
  Mux/1 -> Mux2/1
  Mux2/1 -> re/1
  u/1 -> Delay2/1
  y/1 -> Product/1
  Constant/1 -> Product/2
  Product/1 -> Delay1/1
  Delay3/1 -> Mux/2  "-y(t-2)"
  Delay1/1 -> Mux/1, Delay3/1  "-y(t-1)"
  Delay2/1 -> Mux1/1, Delay4/1  "u(t-1)"
